simulink model "kaskadka"  (R2013a)
settings: Solver=ode45  StartTime=0.0  StopTime=20.0  RelTol=1e-3  AbsTol=1e-6
values from neighbouring files (symbols this model uses):
  A = [-a1/A1 0; a1/A2 -a2/A2]    [transmitacje.m]
  a1 = Aw1*sqrt(2*g*h1max)/h1max    [Kaskady.m]    (also in Kaskady2.m; Skoki.m = 2*Wn*ksi(i); symulek1.m = 1; transmitacje.m)
  A2 = 1    [Kaskady.m]    (also in Kaskady2.m; Palmowski.m = -1-A1; transmitacje.m)
  a2 = Aw2*sqrt(2*g*h2max)/h2max    [Kaskady.m]    (also in Kaskady2.m; Skoki.m = 1; transmitacje.m)
  h10 = fwew1/a1    [Kaskady.m]    (also in Kaskady2.m; transmitacje.m)
  h20 = (fwew1+fwew2)/a2    [Kaskady.m]    (also in Kaskady2.m; transmitacje.m)
  t0 = 1    [Kaskady.m]    (also in Kaskady2.m; Skoki.m = 0; symulek1.m; transmitacje.m)
undefined symbols (not defined in the file or in its folder): dfwe, dfwe2, fwe, fwe2
settings Model: Creator=LAB320-1552  LastModifiedBy=LAB320-1552
settings DebuggingCC: SolverPrmCheckMsg=none

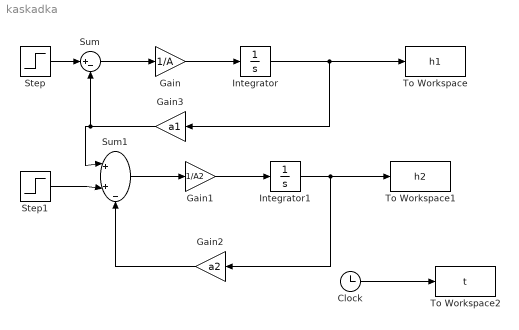
== system kaskadka ==
  Clock : Clock
  Gain : Gain  Gain=1/A
  Gain1 : Gain  Gain=1/A2
  Gain2 : Gain  Gain=a2
  Gain3 : Gain  Gain=a1
  Integrator : Integrator  InitialCondition=h10
  Integrator1 : Integrator  InitialCondition=h20
  Step : Step  Time=t0  Before=fwe  After=fwe+dfwe  SampleTime=0
  Step1 : Step  Time=t0  Before=fwe2  After=fwe2+dfwe2  SampleTime=0
  Sum : Sum  Inputs=|+-
  Sum1 : Sum  Inputs=|++-
  To Workspace : ToWorkspace  VariableName=h1  SampleTime=-1
  To Workspace1 : ToWorkspace  VariableName=h2  SampleTime=-1
  To Workspace2 : ToWorkspace  VariableName=t  SampleTime=-1  SaveFormat=Timeseries
  wires:
  Clock/1 -> To Workspace2/1
  Step/1 -> Sum/1
  Integrator/1 -> Gain3/1, To Workspace/1
  Sum/1 -> Gain/1
  Gain/1 -> Integrator/1
  Step1/1 -> Sum1/2
  Gain2/1 -> Sum1/3
  Sum1/1 -> Gain1/1
  Gain1/1 -> Integrator1/1
  Integrator1/1 -> Gain2/1, To Workspace1/1
  Gain3/1 -> Sum1/1, Sum/2
